simulink model "Brown_6DOF_Sim_Wrapper"  (R2025b)
settings: Solver=VariableStepAuto  StartTime=0.0  StopTime=10  RelTol=1e-3
values from neighbouring files (symbols this model uses):
  controller_sample_time = 0.01    [Brown_6DOF_Init_main.m]    (also in Full_Sim_Init.m; HW356_simple_demos_live_source.m; Init_Main.m)
  gains = apply_default_controller_gains()    [HW34_sensors_rootlocus_live_source.m]
  sensor_sample_time = controller_sample_time    (= 0.01)    [Brown_6DOF_Init_main.m]    (also in Full_Sim_Init.m; Init_Main.m)
undefined symbols (not defined in the file or in its folder): base_set_point, cmd_profile, DiscIntNeverNeededParam, sat, sensors, truth_ic
libraries: Brown_Flight_Controls_lib x8
settings Model: Creator=zbrown  LastModifiedBy=zbrown

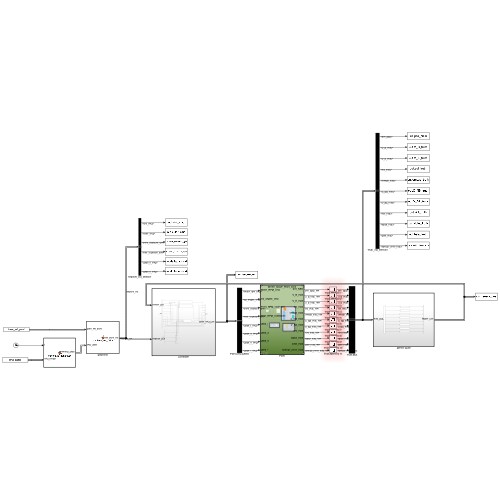
[thumbnail: Simulink's stored preview of the top-level diagram]
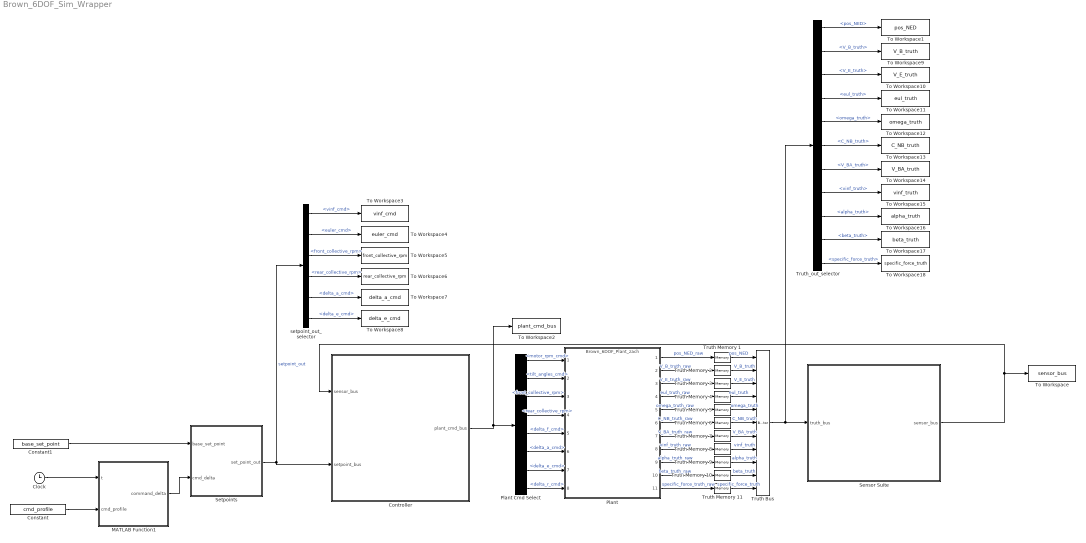
== system Brown_6DOF_Sim_Wrapper ==
  Clock : Clock
  Constant : Constant  Value=cmd_profile  OutDataTypeStr=Bus: CmdProfileBus
  Constant1 : Constant  Value=base_set_point  OutDataTypeStr=Bus: BaseSetPointBus
  Controller : Subsystem  TreatAsAtomicUnit=on  SystemSampleTime=controller_sample_time
  MATLAB Function1 : MATLAB Function  TreatAsAtomicUnit=on
  Plant : ModelReference  ModelNameDialog=Brown_6DOF_Plant_zach  SimulationMode=Normal  ModelReferenceVersion=1.33
  Plant Cmd Select : BusSelector  OutputSignals=motor_rpm_cmd,tilt_angles_cmd,front_collective_rpm,rear_collective_rpm,delta_f_cmd,delta_a_cmd,delta_e_cmd,delta_r_cmd
  Sensor Suite : Subsystem  TreatAsAtomicUnit=on  SystemSampleTime=sensor_sample_time
  Setpoints : MATLAB Function  TreatAsAtomicUnit=on
  To Workspace : ToWorkspace  VariableName=sensor_bus  SaveFormat=Structure With Time  SampleTime=-1
  To Workspace1 : ToWorkspace  VariableName=pos_NED  SaveFormat=Structure With Time  SampleTime=-1
  To Workspace10 : ToWorkspace  VariableName=V_E_truth  SaveFormat=Structure With Time  SampleTime=-1
  To Workspace11 : ToWorkspace  VariableName=eul_truth  SaveFormat=Structure With Time  SampleTime=-1
  To Workspace12 : ToWorkspace  VariableName=omega_truth  SaveFormat=Structure With Time  SampleTime=-1
  To Workspace13 : ToWorkspace  VariableName=C_NB_truth  SaveFormat=Structure With Time  SampleTime=-1
  To Workspace14 : ToWorkspace  VariableName=V_BA_truth  SaveFormat=Structure With Time  SampleTime=-1
  To Workspace15 : ToWorkspace  VariableName=vinf_truth  SaveFormat=Structure With Time  SampleTime=-1
  To Workspace16 : ToWorkspace  VariableName=alpha_truth  SaveFormat=Structure With Time  SampleTime=-1
  To Workspace17 : ToWorkspace  VariableName=beta_truth  SaveFormat=Structure With Time  SampleTime=-1
  To Workspace18 : ToWorkspace  VariableName=specific_force_truth  SaveFormat=Structure With Time  SampleTime=-1
  To Workspace2 : ToWorkspace  VariableName=plant_cmd_bus  SaveFormat=Structure With Time  SampleTime=-1
  To Workspace3 : ToWorkspace  VariableName=vinf_cmd  SaveFormat=Structure With Time  SampleTime=-1
  To Workspace4 : ToWorkspace  VariableName=euler_cmd  SaveFormat=Structure With Time  SampleTime=-1
  To Workspace5 : ToWorkspace  VariableName=front_collective_rpm  SaveFormat=Structure With Time  SampleTime=-1
  To Workspace6 : ToWorkspace  VariableName=rear_collective_rpm  SaveFormat=Structure With Time  SampleTime=-1
  To Workspace7 : ToWorkspace  VariableName=delta_a_cmd  SaveFormat=Structure With Time  SampleTime=-1
  To Workspace8 : ToWorkspace  VariableName=delta_e_cmd  SaveFormat=Structure With Time  SampleTime=-1
  To Workspace9 : ToWorkspace  VariableName=V_B_truth  SaveFormat=Structure With Time  SampleTime=-1
  Truth Bus : BusCreator  Inputs=11  OutDataTypeStr=Bus: TruthBus
  Truth Memory 1 : Memory  InitialCondition=truth_ic.pos_NED
  Truth Memory 10 : Memory  InitialCondition=truth_ic.beta_truth
  Truth Memory 11 : Memory  InitialCondition=truth_ic.specific_force_truth
  Truth Memory 2 : Memory  InitialCondition=truth_ic.V_B_truth
  Truth Memory 3 : Memory  InitialCondition=truth_ic.V_E_truth
  Truth Memory 4 : Memory  InitialCondition=truth_ic.eul_truth
  Truth Memory 5 : Memory  InitialCondition=truth_ic.omega_truth
  Truth Memory 6 : Memory  InitialCondition=truth_ic.C_NB_truth
  Truth Memory 7 : Memory  InitialCondition=truth_ic.V_BA_truth
  Truth Memory 8 : Memory  InitialCondition=truth_ic.vinf_truth
  Truth Memory 9 : Memory  InitialCondition=truth_ic.alpha_truth
  Truth_out_selector : BusSelector  OutputSignals=pos_NED,V_B_truth,V_E_truth,eul_truth,omega_truth,C_NB_truth,V_BA_truth,vinf_truth,alpha_truth,beta_truth,specific_force_truth
  setpoint_out_selector : BusSelector  OutputSignals=vinf_cmd,euler_cmd,front_collective_rpm,rear_collective_rpm,delta_a_cmd,delta_e_cmd
  wires:
  Controller/1(plant_cmd_bus) -> To Workspace2/1, Plant Cmd Select/1
  Plant Cmd Select/1 -> Plant/1  "<motor_rpm_cmd>"
  Plant Cmd Select/2 -> Plant/2  "<tilt_angles_cmd>"
  Plant Cmd Select/3 -> Plant/3  "<front_collective_rpm>"
  Plant Cmd Select/4 -> Plant/4  "<rear_collective_rpm>"
  Plant Cmd Select/5 -> Plant/5  "<delta_f_cmd>"
  Plant Cmd Select/6 -> Plant/6  "<delta_a_cmd>"
  Plant Cmd Select/7 -> Plant/7  "<delta_e_cmd>"
  Plant Cmd Select/8 -> Plant/8  "<delta_r_cmd>"
  Plant/1 -> Truth Memory 1/1  "pos_NED_raw"
  Truth Memory 1/1 -> Truth Bus/1  "pos_NED"
  Plant/2 -> Truth Memory 2/1  "V_B_truth_raw"
  Truth Memory 2/1 -> Truth Bus/2  "V_B_truth"
  Plant/3 -> Truth Memory 3/1  "V_E_truth_raw"
  Truth Memory 3/1 -> Truth Bus/3  "V_E_truth"
  Plant/4 -> Truth Memory 4/1  "eul_truth_raw"
  Truth Memory 4/1 -> Truth Bus/4  "eul_truth"
  Plant/5 -> Truth Memory 5/1  "omega_truth_raw"
  Truth Memory 5/1 -> Truth Bus/5  "omega_truth"
  Plant/6 -> Truth Memory 6/1  "C_NB_truth_raw"
  Truth Memory 6/1 -> Truth Bus/6  "C_NB_truth"
  Plant/7 -> Truth Memory 7/1  "V_BA_truth_raw"
  Truth Memory 7/1 -> Truth Bus/7  "V_BA_truth"
  Plant/8 -> Truth Memory 8/1  "vinf_truth_raw"
  Truth Memory 8/1 -> Truth Bus/8  "vinf_truth"
  Plant/9 -> Truth Memory 9/1  "alpha_truth_raw"
  Truth Memory 9/1 -> Truth Bus/9  "alpha_truth"
  Plant/10 -> Truth Memory 10/1  "beta_truth_raw"
  Truth Memory 10/1 -> Truth Bus/10  "beta_truth"
  Plant/11 -> Truth Memory 11/1  "specific_force_truth_raw"
  Truth Memory 11/1 -> Truth Bus/11  "specific_force_truth"
  Truth Bus/1 -> Truth_out_selector/1, Sensor Suite/1(truth_bus)
  Sensor Suite/1(sensor_bus) -> To Workspace/1, Controller/1(sensor_bus)
  Constant1/1 -> Setpoints/1(base_set_point)
  Setpoints/1(set_point_out) -> setpoint_out_selector/1, Controller/2(setpoint_bus)  "setpoint_out"
  MATLAB Function1/1(command_delta) -> Setpoints/2(cmd_delta)
  Clock/1 -> MATLAB Function1/1(t)
  Constant/1 -> MATLAB Function1/2(cmd_profile)
  setpoint_out_selector/5 -> To Workspace7/1  "<delta_a_cmd>"
  setpoint_out_selector/1 -> To Workspace3/1  "<vinf_cmd>"
  setpoint_out_selector/2 -> To Workspace4/1  "<euler_cmd>"
  setpoint_out_selector/6 -> To Workspace8/1  "<delta_e_cmd>"
  setpoint_out_selector/4 -> To Workspace6/1  "<rear_collective_rpm>"
  setpoint_out_selector/3 -> To Workspace5/1  "<front_collective_rpm>"
  Truth_out_selector/1 -> To Workspace1/1  "<pos_NED>"
  Truth_out_selector/2 -> To Workspace9/1  "<V_B_truth>"
  Truth_out_selector/3 -> To Workspace10/1  "<V_E_truth>"
  Truth_out_selector/4 -> To Workspace11/1  "<eul_truth>"
  Truth_out_selector/5 -> To Workspace12/1  "<omega_truth>"
  Truth_out_selector/6 -> To Workspace13/1  "<C_NB_truth>"
  Truth_out_selector/7 -> To Workspace14/1  "<V_BA_truth>"
  Truth_out_selector/8 -> To Workspace15/1  "<vinf_truth>"
  Truth_out_selector/9 -> To Workspace16/1  "<alpha_truth>"
  Truth_out_selector/10 -> To Workspace17/1  "<beta_truth>"
  Truth_out_selector/11 -> To Workspace18/1  "<specific_force_truth>"

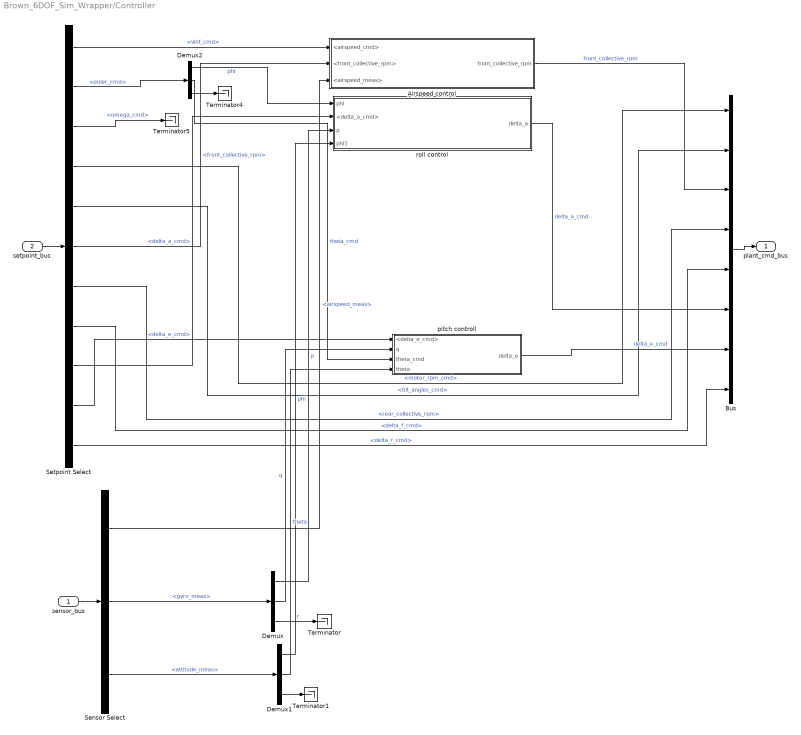
== system Brown_6DOF_Sim_Wrapper/Controller ==
  sensor_bus : Inport
  setpoint_bus : Inport  Port=2
  Airspeed control : Subsystem
  Bus : BusCreator  Inputs=8
  Demux : Demux  Outputs=3
  Demux1 : Demux  Outputs=3
  Demux2 : Demux  Outputs=3
  Sensor Select : BusSelector  OutputSignals=airspeed_meas,gyro_meas,attitude_meas
  Setpoint Select : BusSelector  OutputSignals=vinf_cmd,euler_cmd,omega_cmd,motor_rpm_cmd,tilt_angles_cmd,front_collective_rpm,rear_collective_rpm,delta_f_cmd,delta_a_cmd,delta_e_cmd,delta_r_cmd
  Terminator{,1,4..5} (4 alike) : Terminator
  pitch controll : Subsystem
  roll control : Subsystem
  plant_cmd_bus : Outport
  wires:
  sensor_bus/1 -> Sensor Select/1
  setpoint_bus/1 -> Setpoint Select/1
  Sensor Select/2 -> Demux/1  "<gyro_meas>"
  Setpoint Select/4 -> Bus/1  "<motor_rpm_cmd>"
  Setpoint Select/5 -> Bus/2  "<tilt_angles_cmd>"
  Setpoint Select/8 -> Bus/5  "<delta_f_cmd>"
  Setpoint Select/11 -> Bus/8  "<delta_r_cmd>"
  Bus/1 -> plant_cmd_bus/1
  Sensor Select/3 -> Demux1/1  "<attitude_meas>"
  Demux/3 -> Terminator/1  "r"
  Demux1/3 -> Terminator1/1
  Demux1/2 -> pitch controll/4(theta)  "theta"
  Setpoint Select/6 -> Airspeed control/2(<front_collective_rpm>)  "<front_collective_rpm>"
  Sensor Select/1 -> Airspeed control/3(<airspeed_meas>)  "<airspeed_meas>"
  Airspeed control/1(front_collective_rpm) -> Bus/3  "front_collective_rpm"
  Demux2/1 -> roll control/1(phi)  "phi"
  Setpoint Select/9 -> roll control/2(<delta_a_cmd>)  "<delta_a_cmd>"
  Demux/1 -> roll control/3(p)  "p"
  Demux1/1 -> roll control/4(phi1)  "phi"
  roll control/1(delta_a) -> Bus/6  "delta_a_cmd"
  Setpoint Select/10 -> pitch controll/1(<delta_e_cmd>)  "<delta_e_cmd>"
  Demux/2 -> pitch controll/2(q)  "q"
  pitch controll/1(delta_e) -> Bus/7  "delta_e_cmd"
  Setpoint Select/7 -> Bus/4  "<rear_collective_rpm>"
  Setpoint Select/3 -> Terminator5/1  "<omega_cmd>"
  Demux2/2 -> pitch controll/3(theta_cmd)  "theta_cmd"
  Demux2/3 -> Terminator4/1
  Setpoint Select/1 -> Airspeed control/1(<airspeed_cmd>)  "<vinf_cmd>"
  Setpoint Select/2 -> Demux2/1  "<euler_cmd>"

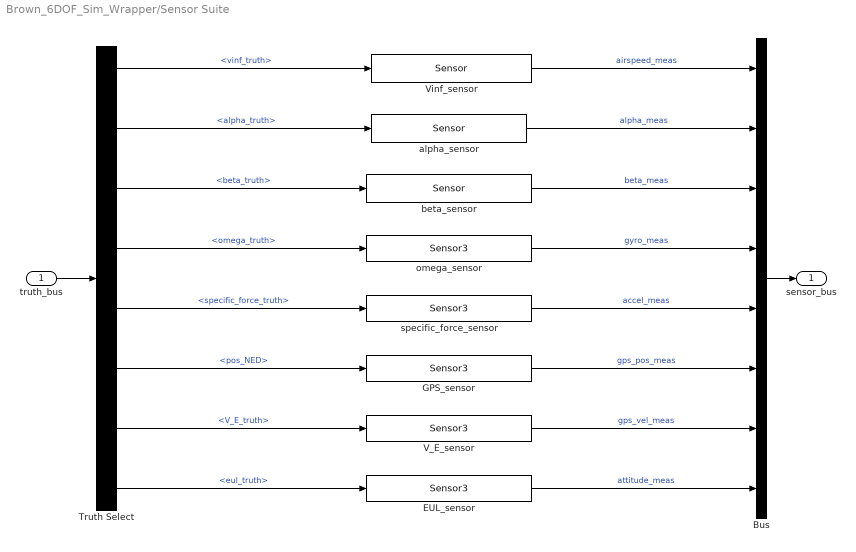
== system Brown_6DOF_Sim_Wrapper/Sensor Suite ==
  truth_bus : Inport
  Bus : BusCreator  Inputs=8
  EUL_sensor : Brown_Flight_Controls_lib/Sensor3  sigma=sensors.eul.sigma  bias3=sensors.eul.bias  Ts=sensors.eul.Ts
  GPS_sensor : Brown_Flight_Controls_lib/Sensor3  sigma=sensors.pos.sigma  bias3=sensors.pos.bias  Ts=sensors.pos.Ts
  Truth Select : BusSelector  OutputSignals=vinf_truth,alpha_truth,beta_truth,omega_truth,specific_force_truth,pos_NED,V_E_truth,eul_truth
  V_E_sensor : Brown_Flight_Controls_lib/Sensor3  sigma=sensors.vel.sigma  bias3=sensors.vel.bias  Ts=sensors.vel.Ts
  Vinf_sensor : Brown_Flight_Controls_lib/Sensor  sigma=sensors.airspeed.sigma  Ts=sensors.airspeed.Ts  bias=sensors.airspeed.bias
  alpha_sensor : Brown_Flight_Controls_lib/Sensor  sigma=sensors.alpha.sigma  Ts=sensors.alpha.Ts  bias=sensors.alpha.bias
  beta_sensor : Brown_Flight_Controls_lib/Sensor  sigma=sensors.beta.sigma  Ts=sensors.beta.Ts  bias=sensors.beta.bias
  omega_sensor : Brown_Flight_Controls_lib/Sensor3  sigma=sensors.omega.sigma  bias3=sensors.omega.bias  Ts=sensors.omega.Ts
  specific_force_sensor : Brown_Flight_Controls_lib/Sensor3  sigma=sensors.accel.sigma  bias3=sensors.accel.bias  Ts=sensors.accel.Ts
  sensor_bus : Outport
  wires:
  truth_bus/1 -> Truth Select/1
  Truth Select/1 -> Vinf_sensor/1  "<vinf_truth>"
  Truth Select/2 -> alpha_sensor/1  "<alpha_truth>"
  Truth Select/3 -> beta_sensor/1  "<beta_truth>"
  Truth Select/4 -> omega_sensor/1  "<omega_truth>"
  Truth Select/5 -> specific_force_sensor/1  "<specific_force_truth>"
  Truth Select/6 -> GPS_sensor/1  "<pos_NED>"
  Truth Select/7 -> V_E_sensor/1  "<V_E_truth>"
  Truth Select/8 -> EUL_sensor/1  "<eul_truth>"
  Vinf_sensor/1 -> Bus/1  "airspeed_meas"
  alpha_sensor/1 -> Bus/2  "alpha_meas"
  beta_sensor/1 -> Bus/3  "beta_meas"
  omega_sensor/1 -> Bus/4  "gyro_meas"
  specific_force_sensor/1 -> Bus/5  "accel_meas"
  GPS_sensor/1 -> Bus/6  "gps_pos_meas"
  V_E_sensor/1 -> Bus/7  "gps_vel_meas"
  EUL_sensor/1 -> Bus/8  "attitude_meas"
  Bus/1 -> sensor_bus/1

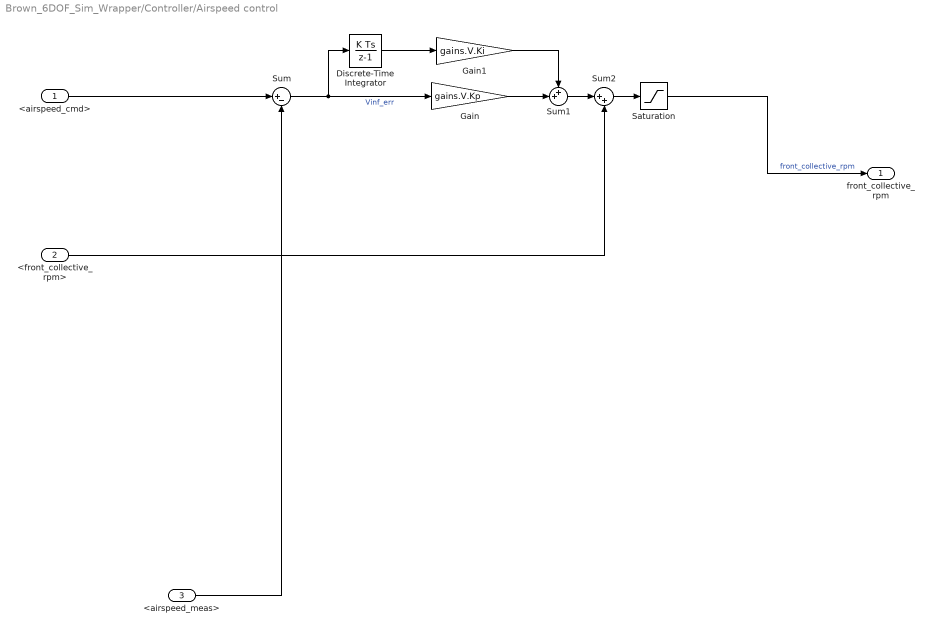
== system Brown_6DOF_Sim_Wrapper/Controller/Airspeed control ==
  <airspeed_cmd> : Inport
  <front_collective_rpm> : Inport  Port=2
  <airspeed_meas> : Inport  Port=3
  Discrete-Time Integrator : DiscreteIntegrator  SampleTime=controller_sample_time  LimitOutput=on  UpperSaturationLimit=5000  LowerSaturationLimit=-5000  ICPrevOutput=DiscIntNeverNeededParam  ICPrevScaledInput=DiscIntNeverNeededParam
  Gain : Gain  Gain=gains.V.Kp
  Gain1 : Gain  Gain=gains.V.Ki
  Saturation : Saturate  UpperLimit=sat.frontcollective.high  LowerLimit=sat.frontcollective.low
  Sum : Sum  Inputs=|+-
  Sum1 : Sum  Inputs=++|
  Sum2 : Sum  Inputs=|++
  front_collective_rpm : Outport
  wires:
  <airspeed_meas>/1 -> Sum/2
  <front_collective_rpm>/1 -> Sum2/2
  Sum2/1 -> Saturation/1
  Sum1/1 -> Sum2/1
  Gain/1 -> Sum1/2
  <airspeed_cmd>/1 -> Sum/1
  Saturation/1 -> front_collective_rpm/1  "front_collective_rpm"
  Gain1/1 -> Sum1/1
  Discrete-Time Integrator/1 -> Gain1/1
  Sum/1 -> Gain/1, Discrete-Time Integrator/1  "Vinf_err"

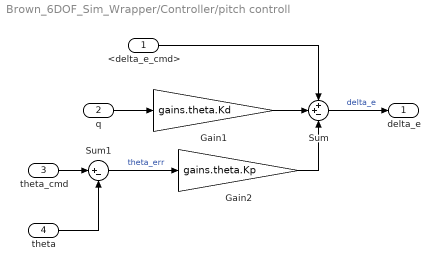
== system Brown_6DOF_Sim_Wrapper/Controller/pitch controll ==
  <delta_e_cmd> : Inport
  q : Inport  Port=2
  theta_cmd : Inport  Port=3
  theta : Inport  Port=4
  Gain1 : Gain  Gain=gains.theta.Kd
  Gain2 : Gain  Gain=gains.theta.Kp
  Sum : Sum  Inputs=++-
  Sum1 : Sum  Inputs=|+-
  delta_e : Outport
  wires:
  q/1 -> Gain1/1
  <delta_e_cmd>/1 -> Sum/1
  Sum/1 -> delta_e/1  "delta_e"
  Gain1/1 -> Sum/2
  Gain2/1 -> Sum/3
  theta/1 -> Sum1/2
  theta_cmd/1 -> Sum1/1
  Sum1/1 -> Gain2/1  "theta_err"

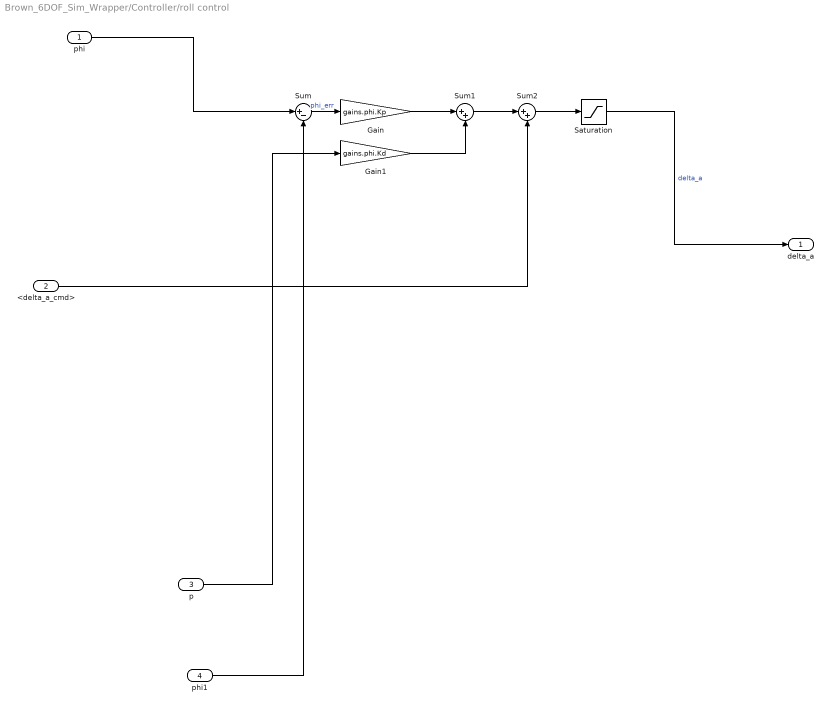
== system Brown_6DOF_Sim_Wrapper/Controller/roll control ==
  phi : Inport
  <delta_a_cmd> : Inport  Port=2
  p : Inport  Port=3
  phi1 : Inport  Port=4
  Gain : Gain  Gain=gains.phi.Kp
  Gain1 : Gain  Gain=gains.phi.Kd
  Saturation : Saturate  UpperLimit=sat.delta_a.high  LowerLimit=sat.delta_a.low
  Sum : Sum  Inputs=|+-
  Sum1 : Sum  Inputs=|++
  Sum2 : Sum  Inputs=|++
  delta_a : Outport
  wires:
  Saturation/1 -> delta_a/1  "delta_a"
  phi/1 -> Sum/1
  <delta_a_cmd>/1 -> Sum2/2
  Sum2/1 -> Saturation/1
  Gain1/1 -> Sum1/2
  Sum/1 -> Gain/1  "phi_err"
  Gain/1 -> Sum1/1
  p/1 -> Gain1/1
  phi1/1 -> Sum/2
  Sum1/1 -> Sum2/1

== matlab function Brown_6DOF_Sim_Wrapper/MATLAB Function1 ==
  data: t input; command_delta output Bus: CommandDeltaBus; cmd_profile input
function command_delta = command_generator(t, cmd_profile)

command_delta = struct( ...
    'd_vinf_cmd', 0.0, ...
    'd_phi_cmd', 0.0, ...
    'd_theta_cmd', 0.0, ...
    'd_p_cmd', 0.0, ...
    'd_q_cmd', 0.0, ...
    'd_r_cmd', 0.0);

if cmd_profile.vinf.enable && cmd_profile.vinf.type == 1
    if t >= cmd_profile.vinf.time
        command_delta.d_vinf_cmd = cmd_profile.vinf.magnitude;
    end
end

if cmd_profile.phi.enable && cmd_profile.phi.type == 1
    if t >= cmd_profile.phi.time
        command_delta.d_phi_cmd = cmd_profile.phi.magnitude;
    end
end

if cmd_profile.theta.enable && cmd_profile.theta.type == 1
    if t >= cmd_profile.theta.time
        command_delta.d_theta_cmd = cmd_profile.theta.magnitude;
    end
end
end

== matlab function Brown_6DOF_Sim_Wrapper/Setpoints ==
  data: base_set_point input; set_point_out output Bus: BaseSetPointBus; cmd_delta input
function set_point_out = combine_set_point(base_set_point, cmd_delta)
%#codegen

set_point_out = base_set_point;

set_point_out.vinf_cmd = base_set_point.vinf_cmd + cmd_delta.d_vinf_cmd;

eul_cmd = base_set_point.euler_cmd(:);
if numel(eul_cmd) ~= 3
    eul_cmd = zeros(3,1);
end
eul_cmd(1) = eul_cmd(1) + cmd_delta.d_phi_cmd;
eul_cmd(2) = eul_cmd(2) + cmd_delta.d_theta_cmd;
set_point_out.euler_cmd = eul_cmd;

set_point_out.omega_cmd = base_set_point.omega_cmd(:) + [ ...
    cmd_delta.d_p_cmd; ...
    cmd_delta.d_q_cmd; ...
    cmd_delta.d_r_cmd];
end
